simulink model "WrongBackTrack"  (R2020b)
settings: Solver=VariableStepAuto  StartTime=0.0  StopTime=10.0  RelTol=1e-3
settings Model: Creator=apple  LastModifiedBy=apple

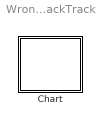
== system WrongBackTrack ==
  Chart : Stateflow chart  TreatAsAtomicUnit=on

== stateflow chart WrongBackTrack/Chart ==
  state A
    en:fprintf("Entry A");
    du:fprintf("During A");
    ex:fprintf("Exit A");
  state B
    en:fprintf("Entry B");
    du:fprintf("During B");
    ex:fprintf("Exit B");
  (default) -> A : {x = 0;}
  A -> (junction 4) [order 1] : [x > -1]{fprintf("Condition Action1");}
  (junction 4) -> (junction 5) : [x > -1]{fprintf("Condition Action3");}
  (junction 5) -> B : [x > 0]{fprintf("Condition Action4");}
  A -> (junction 4) [order 2] : [x > -3]{fprintf("Condition Action2");}
  data: x local
